simulink model "AdaptiveCruiseControl"  (R2021b)
settings: Solver=VariableStepAuto  StartTime=0.0  StopTime=2  RelTol=1e-3
libraries: rllib x1
settings Model: Creator=Hanky  LastModifiedBy=Hanky

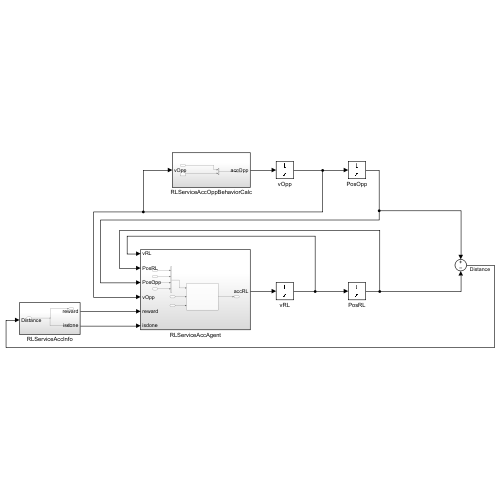
[thumbnail: Simulink's stored preview of the top-level diagram]
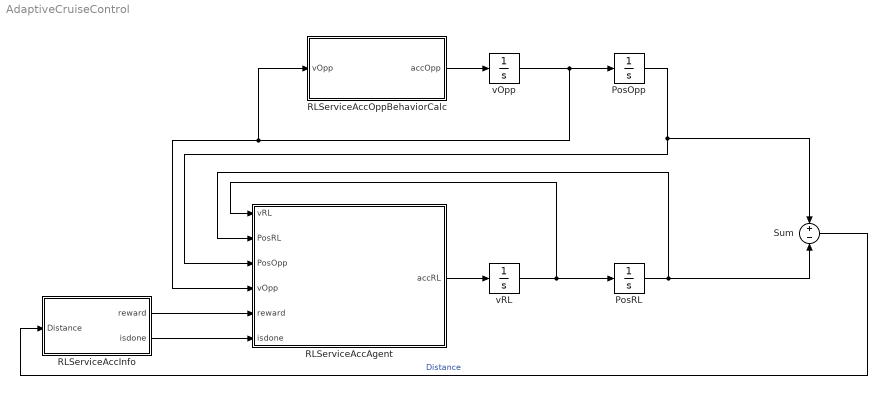
== system AdaptiveCruiseControl ==
  PosOpp : Integrator  InitialCondition=50
  PosRL : Integrator
  RLServiceAccAgent : Subsystem
  RLServiceAccInfo : Subsystem
  RLServiceAccOppBehaviorCalc : Subsystem
  Sum : Sum  Inputs=+-
  vOpp : Integrator
  vRL : Integrator
  wires:
  PosOpp/1 -> RLServiceAccAgent/3(PosOpp), Sum/1
  vRL/1 -> PosRL/1, RLServiceAccAgent/1(vRL)
  vOpp/1 -> RLServiceAccOppBehaviorCalc/1(vOpp), RLServiceAccAgent/4(vOpp), PosOpp/1
  PosRL/1 -> RLServiceAccAgent/2(PosRL), Sum/2
  Sum/1 -> RLServiceAccInfo/1(Distance)  "Distance"
  RLServiceAccInfo/1(reward) -> RLServiceAccAgent/5(reward)
  RLServiceAccInfo/2(isdone) -> RLServiceAccAgent/6(isdone)
  RLServiceAccAgent/1(accRL) -> vRL/1
  RLServiceAccOppBehaviorCalc/1(accOpp) -> vOpp/1

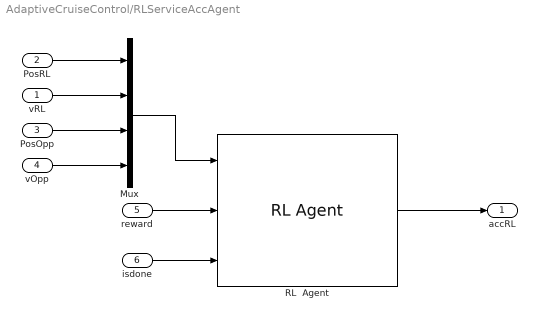
== system AdaptiveCruiseControl/RLServiceAccAgent ==
  vRL : Inport
  PosRL : Inport  Port=2
  PosOpp : Inport  Port=3
  vOpp : Inport  Port=4
  reward : Inport  Port=5
  isdone : Inport  Port=6
  Mux : Mux
  RL  Agent : rllib/RL Agent  Agent=agentObj  ExternalActionAsInput=off  ProvideCumRwd=off  TreatAsDirectFeedthrough=on
  accRL : Outport
  wires:
  Mux/1 -> RL  Agent/1
  vRL/1 -> Mux/2
  isdone/1 -> RL  Agent/3
  RL  Agent/1 -> accRL/1
  reward/1 -> RL  Agent/2
  PosRL/1 -> Mux/1
  vOpp/1 -> Mux/4
  PosOpp/1 -> Mux/3

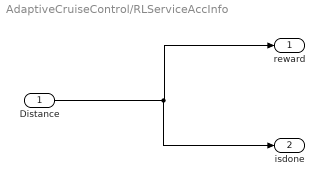
== system AdaptiveCruiseControl/RLServiceAccInfo ==
  Distance : Inport
  reward : Outport
  isdone : Outport  Port=2
  wires:
  Distance/1 -> isdone/1, reward/1

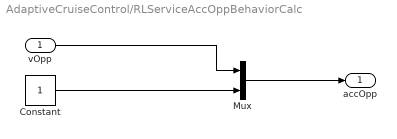
== system AdaptiveCruiseControl/RLServiceAccOppBehaviorCalc ==
  vOpp : Inport
  Constant : Constant
  Mux : Mux  Inputs=2
  accOpp : Outport
  wires:
  Constant/1 -> Mux/2
  vOpp/1 -> Mux/1
  Mux/1 -> accOpp/1
